simulink model "All_Car_Models"  (R2018b)
settings: Solver=VariableStepAuto  StartTime=0.0  StopTime=10.0  RelTol=1e-3
values from neighbouring files (symbols this model uses):
  a = 1.25    [SetCoefficients_FC.m]
  amplitude = 0.01    [SetCoefficients_FC.m]
  b = 1.4    [SetCoefficients_FC.m]
  c = 1.3    [SetCoefficients_FC.m]
  csc = 600    [SetCoefficients_FC.m]
  cse = 1200    [SetCoefficients_FC.m]
  d = 1.7    [SetCoefficients_FC.m]
  delay = (a+b)/v    [setSpeed.m]
  Fre_r = Fre*2*pi    [setSpeed.m]
  g = 9.81    [SetCoefficients_FC.m]
  HumpHight = 2    [SetCoefficients_FC.m]
  HumpLegnth = 20    [SetCoefficients_FC.m]
  I = 600    [SetCoefficients_FC.m]
  I_phi = 1000    [SetCoefficients_FC.m]
  I_theta = 600    [SetCoefficients_FC.m]
  ks =     [SetCoefficients.m]    (also in SetCoefficients_FC.m = 20000)
  ksSteel = 6.6e9    (= 6600000000)    [SetCoefficients_FC.m]
  ksstiff = 4e5    (= 400000)    [SetCoefficients_FC.m]
  kt =     [SetCoefficients.m]    (also in SetCoefficients_FC.m = 140000)
  m1 = 250    [SetCoefficients.m]    (also in SetCoefficients_FC.m)
  m2 =     [SetCoefficients.m]    (also in SetCoefficients_FC.m = 20)
  mb = 1000    [SetCoefficients_FC.m]
  mbh = mb/2    (= 500)    [SetCoefficients_FC.m]
  v_hump = v    [setSpeed.m]
  x1 = 0.2    [SetCoefficients_FC.m]
  x2 = 0.25    [SetCoefficients_FC.m]
  xt_Lim = 0.1    [SetCoefficients_FC.m]
(part 1 of 2)
settings Model: Creator=joebe  LastModifiedBy=joebe

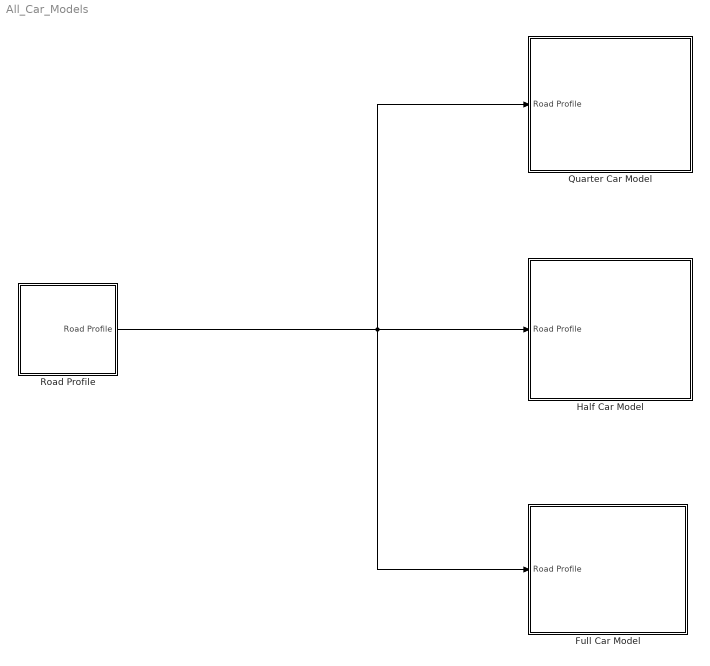
== system All_Car_Models ==
  Full Car Model : Subsystem
  Half Car Model : Subsystem
  Quarter Car Model : Subsystem
  Road Profile : Subsystem
  wires:
  Road Profile/1(Road Profile) -> Quarter Car Model/1(Road Profile), Full Car Model/1(Road Profile), Half Car Model/1(Road Profile)

== system All_Car_Models/Full Car Model ==
  Road Profile : Inport
  Bus Selector : BusSelector  OutputSignals=Body Vertical Motion.COM Displacement,Body Vertical Motion.COM Velocity,body pitch motion.Pitch Angle,body pitch motion.Pitch Velocity,Body Pitch motion.Roll Angle,Body Pitch motion.Roll Velocity
  Bus Selector1 : BusSelector  OutputSignals=Front Left Body Motion.Front Left Displacement,Front Right Body Motion.Front Right Displacement,Rear Left Body Motion.Rear Left Displacement,Rear Right Body Motion.Rear Right Displacement
  COM/Road displacement : Scope  NumInputPorts=2
  Full Car Model : Subsystem
  Pitch Angle : Scope
  Pitch Velocity : Scope
  Roll Angle : Scope
  Roll Velocity : Scope
  Tyre/COM displacements : Scope  NumInputPorts=5
  Vertical Displacement : Scope
  Vertical Velocity : Scope
  wires:
  Bus Selector1/2 -> Tyre/COM displacements/2  "<Front Right Displacement>"
  Bus Selector/3 -> Pitch Angle/1  "<Pitch Angle>"
  Full Car Model/1(Body Motion) -> Bus Selector/1
  Bus Selector/6 -> Roll Velocity/1  "<Roll Velocity>"
  Bus Selector/5 -> Roll Angle/1  "<Roll Angle>"
  Bus Selector/1 -> Vertical Displacement/1, Tyre/COM displacements/5, COM/Road displacement/1  "<COM Displacement>"
  Bus Selector/2 -> Vertical Velocity/1  "<COM Velocity>"
  Road Profile/1 -> Full Car Model/1(Road Profile), COM/Road displacement/2
  Bus Selector1/1 -> Tyre/COM displacements/1  "<Front Left Displacement>"
  Bus Selector1/3 -> Tyre/COM displacements/3  "<Rear Left Displacement>"
  Bus Selector/4 -> Pitch Velocity/1  "<Pitch Velocity>"
  Full Car Model/2(Body Section Motion) -> Bus Selector1/1
  Bus Selector1/4 -> Tyre/COM displacements/4  "<Rear Right Displacement>"

== system All_Car_Models/Half Car Model ==
  Road Profile : Inport
  1/2 Car Model : Subsystem
  1/2 Car Model Improved : Subsystem
  Body displacements : Scope  NumInputPorts=3
  Body displacements Improved model : Scope  NumInputPorts=3
  COM Body comparrison : Scope  NumInputPorts=2
  Demux{,1,3..4} (4 alike) : Demux
  wires:
  Demux1/3 -> Body displacements/2  "Rear Body displacement"
  Demux3/1 -> Body displacements Improved model/3, COM Body comparrison/2  "COM Displacement Improved Model"
  1/2 Car Model/2(Body Section motions) -> Demux1/1
  Demux/1 -> COM Body comparrison/1, Body displacements/3  "COM Displcameent Original Model"
  1/2 Car Model Improved/2(Body Section motions) -> Demux4/1
  Demux4/1 -> Body displacements Improved model/1  "Front Body Displacement"
  Road Profile/1 -> 1/2 Car Model/1(Road Profile), 1/2 Car Model Improved/1(Road Profile)
  1/2 Car Model Improved/1(Body Motion. (sb.sbd.theta,thetad)) -> Demux3/1
  Demux4/3 -> Body displacements Improved model/2  "Rear Body displacement"
  1/2 Car Model/1(Body Motion) -> Demux/1
  Demux1/1 -> Body displacements/1  "Front Body Displacement"

== system All_Car_Models/Quarter Car Model ==
  Road Profile : Inport
  Body Displacement : Scope
  Body Velocity : Scope
  Body Wheel and Road Displacement : Scope  NumInputPorts=3
  Demux : Demux  Outputs=2
  Demux1 : Demux  Outputs=2
  Quarter Car Model : Subsystem
  Wheel Displacement : Scope
  Wheel Velocity : Scope
  wires:
  Demux/2 -> Body Velocity/1  "Body Velcoity"
  Demux1/1 -> Body Wheel and Road Displacement/3, Wheel Displacement/1  "Wheel Displacement"
  Demux1/2 -> Wheel Velocity/1  "Wheel Velocity"
  Road Profile/1 -> Body Wheel and Road Displacement/2, Quarter Car Model/1(Road profile)
  Demux/1 -> Body Wheel and Road Displacement/1, Body Displacement/1  "Body Displacement"
  Quarter Car Model/1(Body Motion) -> Demux/1
  Quarter Car Model/2(Wheel Motion) -> Demux1/1

== system All_Car_Models/Road Profile ==
  Constant : Constant  Value=0
  Delay : TransportDelay  BufferSize=3072
  Delay1 : TransportDelay  BufferSize=3072
  Humpback bridge : Subsystem  mask{h=HumpHight, L=HumpLegnth, v=v_hump}
      mask prompts: h "humpback height (m)"; L "humpback length (m)"; v "vehicle speed (m/s)"
  Sine Wave : Sin  Amplitude=amplitude  Frequency=Fre_r  SampleTime=0
  Step Drop : Step  Time=2  After=-5  SampleTime=0
  Step Increase : Step  Time=2  SampleTime=0
  Road Profile : Outport
  wires:
  Humpback bridge/1(r) -> Delay1/1
  Sine Wave/1 -> Delay/1
  Delay1/1 -> Road Profile/1  "Road Profile"

== system All_Car_Models/Full Car Model/Full Car Model ==
  Road Profile : Inport
  Bus Creator : BusCreator  Inputs=4
  Bus Selector : BusSelector  OutputSignals=Front Left Body Motion,Rear Left Body Motion,Front Right Body Motion,Rear Right Body Motion
  Delay from front to rear wheels : TransportDelay  DelayTime=delay  BufferSize=3072
  Front Left Wheel Suspension model : Subsystem
  Front Right Suspension model : Subsystem
  Full Car Body Model : Subsystem
  Rear Left Wheel Suspension model : Subsystem
  Rear Right Suspension model : Subsystem
  Body Motion : Outport
  Body Section Motion : Outport  Port=2
  wires:
  Full Car Body Model/1(Body Motion) -> Body Motion/1
  Delay from front to rear wheels/1 -> Rear Right Suspension model/2(Road Profile), Rear Left Wheel Suspension model/2(Road Profile)
  Road Profile/1 -> Delay from front to rear wheels/1, Front Left Wheel Suspension model/2(Road Profile), Front Right Suspension model/2(Road Profile)
  Bus Selector/1 -> Front Left Wheel Suspension model/1(Body Motion)  "<Front Left Body Motion>"
  Front Left Wheel Suspension model/1(Front Left Suspension Force) -> Bus Creator/1  "Front Left  Suspension Force"
  Rear Right Suspension model/1(Rear Right Suspension Force) -> Bus Creator/3  "Rear Right  Suspension Force"
  Front Right Suspension model/1(Front Right Suspension Force) -> Bus Creator/4  "Front Right  Suspension Force"
  Bus Selector/3 -> Front Right Suspension model/1(Body Motion)  "<Front Right Body Motion>"
  Full Car Body Model/2(Body Section Motion) -> Bus Selector/1, Body Section Motion/1  "Body Section Motions"
  Bus Selector/2 -> Rear Left Wheel Suspension model/1(Body Motion)  "<Rear Left Body Motion>"
  Rear Left Wheel Suspension model/1(Rear Left Suspension Force) -> Bus Creator/2  "Rear Left  Suspension Force"
  Bus Selector/4 -> Rear Right Suspension model/1(Body Motion)  "<Rear Right Body Motion>"
  Bus Creator/1 -> Full Car Body Model/1(Suspention Forces)

== system All_Car_Models/Half Car Model/1//2 Car Model ==
  Road Profile : Inport
  1/2 car body model : Subsystem
  Delay from front to rear wheel : TransportDelay  DelayTime=delay  BufferSize=3072
  Front Wheel Suspention model : Subsystem
  Mux : Mux  Inputs=2
  Rear Wheel Suspention model : Subsystem
  Body Motion : Outport
  Body Section motions : Outport  Port=2
  wires:
  1/2 car body model/3(Rear Body Motion) -> Rear Wheel Suspention model/2(Body Motion), Mux/2  "Rear Body Motion"
  Front Wheel Suspention model/1(Front Suspention Force) -> 1/2 car body model/1(Front Suspention Force)  "Front Suspention Force"
  Rear Wheel Suspention model/1(Rear Suspention Force) -> 1/2 car body model/2(Rear Suspention Force)  "Rear Suspention Force"
  1/2 car body model/1(Front Body Motion) -> Front Wheel Suspention model/1(Body Motion), Mux/1  "Front Body Motion"
  1/2 car body model/2(Body Motion) -> Body Motion/1
  Road Profile/1 -> Front Wheel Suspention model/2(Road Profile), Delay from front to rear wheel/1
  Mux/1 -> Body Section motions/1
  Delay from front to rear wheel/1 -> Rear Wheel Suspention model/1(Road Profile)

== system All_Car_Models/Half Car Model/1//2 Car Model Improved ==
  note: Rear
  Road Profile : Inport
  1/2 car body model : Subsystem
  Delay from front to rear wheel2 : TransportDelay  DelayTime=delay  BufferSize=3072
  Front Wheel Suspension model : Subsystem
  Mux : Mux  Inputs=2
  Rear Wheel Suspension model : Subsystem
  Body Motion. (sb.sbd.theta,thetad) : Outport
  Body Section motions : Outport  Port=2
  wires:
  1/2 car body model/3(Rear Body Motion) -> Rear Wheel Suspension model/2(Body Motion), Mux/2  "Rear Body Motion"
  Front Wheel Suspension model/1(Fs) -> 1/2 car body model/1(Front Suspension Force)  "Front Suspension Force"
  Rear Wheel Suspension model/1(Fs) -> 1/2 car body model/2(Rear Suspension Force)  "Rear Suspension Force"
  1/2 car body model/1(Front Body Motion) -> Mux/1, Front Wheel Suspension model/1(Body Motion)  "Front Body Motion"
  1/2 car body model/2(Body Motion) -> Body Motion. (sb.sbd.theta,thetad)/1  "Body Motion. (sb.sbd.theta,thetad)"
  Road Profile/1 -> Delay from front to rear wheel2/1, Front Wheel Suspension model/2(Road Profile)
  Mux/1 -> Body Section motions/1
  Delay from front to rear wheel2/1 -> Rear Wheel Suspension model/1(Road Profile)

== system All_Car_Models/Quarter Car Model/Quarter Car Model ==
  Road profile : Inport
  Body Model : Subsystem
  Suspention Model : Subsystem
  Wheel Model : Subsystem
  Body Motion : Outport
  Wheel Motion : Outport  Port=2
  wires:
  Suspention Model/1(Suspention Force) -> Body Model/1("Suspention Force "), Wheel Model/2(Suspention force)  "Suspention Force"
  Wheel Model/1(Wheel Motion) -> Wheel Motion/1, Suspention Model/1(Wheel Motion)  "Wheel Motion"
  Body Model/1(Body Motion) -> Body Motion/1, Suspention Model/2(Body Motion)  "Body Motion"
  Road profile/1 -> Wheel Model/1(Road Profile)  "Road Profile"

== system All_Car_Models/Road Profile/Humpback bridge ==
  Add : Sum  Inputs=+-
  Constant : Constant  Value=h/2
  Product : Product
  Product1 : Product
  Sine Wave : Sin  Amplitude=h/2  Frequency=2*pi*v_hump/L  Phase=pi/2  SampleTime=0
  Step : Step  Time=0  SampleTime=0
  Step1 : Step  Time=L/v_hump  Before=1  After=0  SampleTime=0
  r : Outport
  wires:
  Constant/1 -> Add/1
  Sine Wave/1 -> Add/2
  Add/1 -> Product/1
  Step/1 -> Product/2
  Product/1 -> Product1/1
  Step1/1 -> Product1/2
  Product1/1 -> r/1

== system All_Car_Models/Full Car Model/Full Car Model/Front Left Wheel Suspension model ==
  Body Motion : Inport
  Road Profile : Inport  Port=2
  Suspention Model : Subsystem
  Wheel Model : Subsystem
  Front Left Suspension Force : Outport
  wires:
  Wheel Model/1(Wheel Motion) -> Suspention Model/1(Wheel Motion)  "s2.s2d"
  Road Profile/1 -> Wheel Model/2(Road Profile)
  Suspention Model/1(Suspension Force) -> Front Left Suspension Force/1, Wheel Model/1(Suspension force)
  Body Motion/1 -> Suspention Model/2(Body Motion)

== system All_Car_Models/Full Car Model/Full Car Model/Front Right Suspension model ==
  Body Motion : Inport
  Road Profile : Inport  Port=2
  Suspension Model : Subsystem
  Wheel Model : Subsystem
  Front Right Suspension Force : Outport
  wires:
  Wheel Model/1(Wheel Motion) -> Suspension Model/1(Wheel Motion)  "s2.s2d"
  Road Profile/1 -> Wheel Model/2(Road Profile)
  Suspension Model/1(Suspension Force) -> Front Right Suspension Force/1, Wheel Model/1(Suspension force)
  Body Motion/1 -> Suspension Model/2(Body Motion)

== system All_Car_Models/Full Car Model/Full Car Model/Full Car Body Model ==
  Suspention Forces : Inport
  Bus Creator : BusCreator  Inputs=3
  Bus Creator1 : BusCreator  Inputs=4
  Bus Selector : BusSelector  OutputSignals=|
      | Front Right 
      | Suspension Force,Front Left 
      | Suspension Force,Rear Right 
      | Suspension Force,Rear Left 
      | Suspension Force
  Car Pitch Motion : Subsystem
  Car Roll Motion1 : Subsystem
  Car Vertical Motion : Subsystem
  Front Left Body Motion : Subsystem
  "Front Right Body Motion " : Subsystem
  Rear Left Body Motion : Subsystem
  Rear Right Body Motion : Subsystem
  Body Motion : Outport
  Body Section Motion : Outport  Port=2
  wires:
  Bus Selector/1 -> Car Roll Motion1/1(Front Right Suspention force), Car Pitch Motion/1(Front Right Suspention force), Car Vertical Motion/1(Front Right Suspention force)  "<Front Right  Suspension Force>"
  Bus Selector/2 -> Car Roll Motion1/2(Front Left Suspention force), Car Pitch Motion/2(Front Left Suspention force), Car Vertical Motion/2(Front Left Suspention force)  "<Front Left  Suspension Force>"
  Bus Selector/3 -> Car Roll Motion1/3(Rear Right Suspention force), Car Pitch Motion/3(Rear Right Suspention force), Car Vertical Motion/3(Rear Right Suspention force)  "<Rear Right  Suspension Force>"
  Car Vertical Motion/1(Body Vertical Motion) -> Bus Creator/1, Rear Right Body Motion/1(Body Vertical Motion), Rear Left Body Motion/1(Body Vertical Motion), "Front Right Body Motion "/1(Body Vertical Motion), Front Left Body Motion/1(Body Vertical Motion)
  Bus Selector/4 -> Car Roll Motion1/4(Rear Left Suspention force), Car Pitch Motion/4(Rear Left Suspention force), Car Vertical Motion/4(Rear Left Suspention force)  "<Rear Left  Suspension Force>"
  Car Roll Motion1/1(Body Roll Motion) -> Front Left Body Motion/3(Body Roll Motion), "Front Right Body Motion "/3(Body Roll Motion), Rear Left Body Motion/3(Body Roll Motion), Bus Creator/3, Rear Right Body Motion/3(Body Roll Motion)
  Car Pitch Motion/1(body pitch motion) -> Front Left Body Motion/2(Body Pitch Motion), "Front Right Body Motion "/2(Body Pitch Motion), Bus Creator/2, Rear Right Body Motion/2(Body Pitch Motion), Rear Left Body Motion/2(Body Pitch Motion)
  Bus Creator/1 -> Body Motion/1
  Bus Creator1/1 -> Body Section Motion/1
  Front Left Body Motion/1(Front Left Body Motion) -> Bus Creator1/1
  "Front Right Body Motion "/1(Front Right Body Motion) -> Bus Creator1/2
  Rear Left Body Motion/1(Rear Left Body Motion) -> Bus Creator1/3
  Rear Right Body Motion/1(Rear Right Body Motion) -> Bus Creator1/4
  Suspention Forces/1 -> Bus Selector/1

== system All_Car_Models/Full Car Model/Full Car Model/Rear Left Wheel Suspension model ==
  Body Motion : Inport
  Road Profile : Inport  Port=2
  Suspension Model : Subsystem
  Wheel Model : Subsystem
  Rear Left Suspension Force : Outport
  wires:
  Wheel Model/1(Wheel Motion) -> Suspension Model/1(Wheel Motion)  "s2.s2d"
  Road Profile/1 -> Wheel Model/2(Road Profile)
  Suspension Model/1(Suspension Force) -> Rear Left Suspension Force/1, Wheel Model/1(Suspension force)
  Body Motion/1 -> Suspension Model/2(Body Motion)

== system All_Car_Models/Full Car Model/Full Car Model/Rear Right Suspension model ==
  Body Motion : Inport
  Road Profile : Inport  Port=2
  Suspention Model : Subsystem
  Wheel Model : Subsystem
  Rear Right Suspension Force : Outport
  wires:
  Wheel Model/1(Wheel Motion) -> Suspention Model/1(Wheel Motion)  "s2.s2d"
  Road Profile/1 -> Wheel Model/2(Road Profile)
  Suspention Model/1(Suspension Force) -> Rear Right Suspension Force/1, Wheel Model/1(Suspension force)
  Body Motion/1 -> Suspention Model/2(Body Motion)

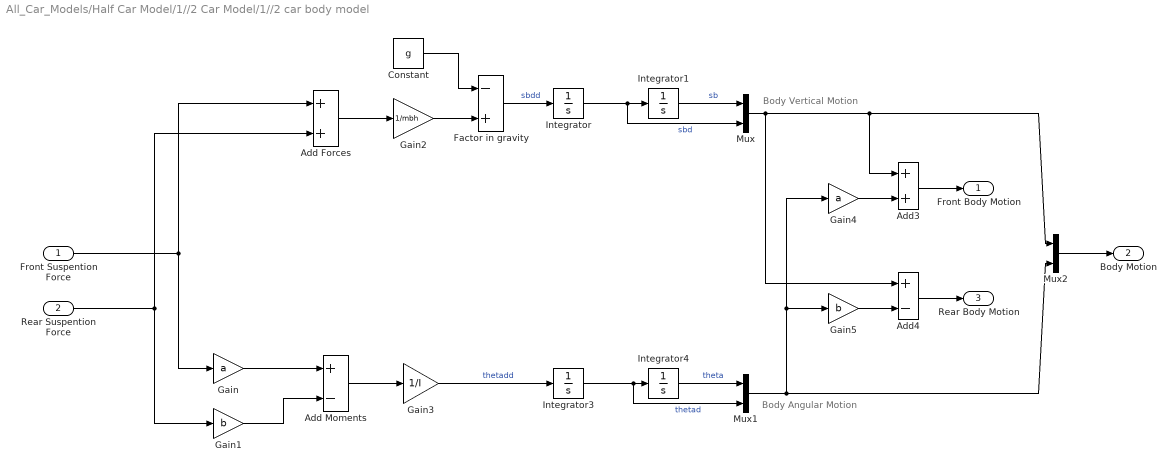
== system All_Car_Models/Half Car Model/1//2 Car Model/1//2 car body model ==
  note: Body Angular Motion
  note: Body Vertical Motion
  Front Suspention Force : Inport
  Rear Suspention Force : Inport  Port=2
  Add Forces : Sum
  Add Moments : Sum  Inputs=+-
  Add3 : Sum
  Add4 : Sum  Inputs=+-
  Constant : Constant  Value=g
  Factor in gravity : Sum  Inputs=-+
  Gain : Gain  Gain=a
  Gain1 : Gain  Gain=b
  Gain2 : Gain  Gain=1/mbh
  Gain3 : Gain  Gain=1/I
  Gain4 : Gain  Gain=a
  Gain5 : Gain  Gain=b
  Integrator : Integrator
  Integrator1 : Integrator  InitialCondition=-0.142
  Integrator3 : Integrator
  Integrator4 : Integrator  InitialCondition=-6e-3
  Mux : Mux  Inputs=2
  Mux1 : Mux  Inputs=2
  Mux2 : Mux  Inputs=2
  Front Body Motion : Outport
  Body Motion : Outport  Port=2
  Rear Body Motion : Outport  Port=3
  wires:
  Add Forces/1 -> Gain2/1
  Mux1/1 -> Gain4/1, Gain5/1, Mux2/2
  Integrator3/1 -> Mux1/2, Integrator4/1  "thetad"
  Add Moments/1 -> Gain3/1
  Gain3/1 -> Integrator3/1  "thetadd"
  Mux2/1 -> Body Motion/1
  Gain2/1 -> Factor in gravity/2
  Mux/1 -> Add4/1, Add3/1, Mux2/1
  Gain4/1 -> Add3/2
  Gain/1 -> Add Moments/1
  Integrator4/1 -> Mux1/1  "theta"
  Integrator/1 -> Mux/2, Integrator1/1  "sbd"
  Rear Suspention Force/1 -> Add Forces/2, Gain1/1
  Front Suspention Force/1 -> Gain/1, Add Forces/1
  Integrator1/1 -> Mux/1  "sb"
  Gain1/1 -> Add Moments/2
  Add3/1 -> Front Body Motion/1
  Gain5/1 -> Add4/2
  Constant/1 -> Factor in gravity/1
  Factor in gravity/1 -> Integrator/1  "sbdd"
  Add4/1 -> Rear Body Motion/1

== system All_Car_Models/Half Car Model/1//2 Car Model/Front Wheel Suspention model ==
  Body Motion : Inport
  Road Profile : Inport  Port=2
  Suspention Model : Subsystem
  Wheel Model : Subsystem
  Front Suspention Force : Outport
  wires:
  Wheel Model/1(Wheel Motion) -> Suspention Model/1(Wheel Motion)
  Road Profile/1 -> Wheel Model/2(Road Profile)
  Suspention Model/1(Suspention Force) -> Front Suspention Force/1, Wheel Model/1(Suspention force)
  Body Motion/1 -> Suspention Model/2(Body Motion)

== system All_Car_Models/Half Car Model/1//2 Car Model/Rear Wheel Suspention model ==
  Road Profile : Inport
  Body Motion : Inport  Port=2
  Suspention Model : Subsystem
  Wheel Model : Subsystem
  Rear Suspention Force : Outport
  wires:
  Wheel Model/1(Wheel Motion) -> Suspention Model/1(Wheel Motion)  "s2.s2d"
  Road Profile/1 -> Wheel Model/2(Road Profile)
  Suspention Model/1(Suspention Force) -> Rear Suspention Force/1, Wheel Model/1(Suspention force)
  Body Motion/1 -> Suspention Model/2(Body Motion)

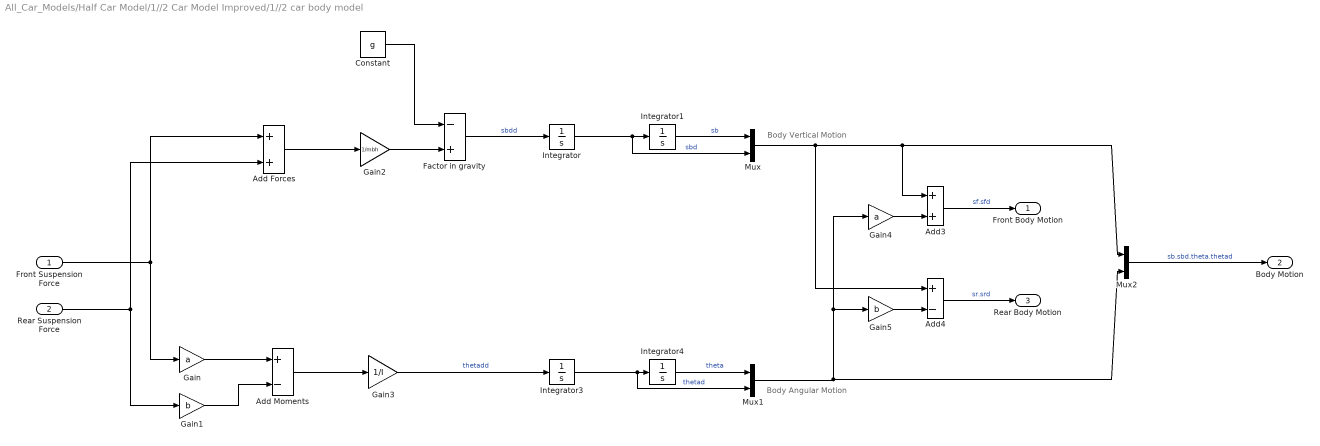
== system All_Car_Models/Half Car Model/1//2 Car Model Improved/1//2 car body model ==
  note: Body Angular Motion
  note: Body Vertical Motion
  Front Suspension Force : Inport
  Rear Suspension Force : Inport  Port=2
  Add Forces : Sum
  Add Moments : Sum  Inputs=+-
  Add3 : Sum
  Add4 : Sum  Inputs=+-
  Constant : Constant  Value=g
  Factor in gravity : Sum  Inputs=-+
  Gain : Gain  Gain=a
  Gain1 : Gain  Gain=b
  Gain2 : Gain  Gain=1/mbh
  Gain3 : Gain  Gain=1/I
  Gain4 : Gain  Gain=a
  Gain5 : Gain  Gain=b
  Integrator : Integrator
  Integrator1 : Integrator  InitialCondition=-0.142
  Integrator3 : Integrator
  Integrator4 : Integrator  InitialCondition=-6e-3
  Mux : Mux  Inputs=2
  Mux1 : Mux  Inputs=2
  Mux2 : Mux  Inputs=2
  Front Body Motion : Outport
  Body Motion : Outport  Port=2
  Rear Body Motion : Outport  Port=3
  wires:
  Add Forces/1 -> Gain2/1
  Mux1/1 -> Gain4/1, Gain5/1, Mux2/2
  Integrator3/1 -> Mux1/2, Integrator4/1  "thetad"
  Add Moments/1 -> Gain3/1
  Gain3/1 -> Integrator3/1  "thetadd"
  Mux2/1 -> Body Motion/1  "sb.sbd.theta.thetad"
  Gain2/1 -> Factor in gravity/2
  Mux/1 -> Add4/1, Add3/1, Mux2/1
  Gain4/1 -> Add3/2
  Gain/1 -> Add Moments/1
  Integrator4/1 -> Mux1/1  "theta"
  Integrator/1 -> Mux/2, Integrator1/1  "sbd"
  Rear Suspension Force/1 -> Add Forces/2, Gain1/1
  Front Suspension Force/1 -> Gain/1, Add Forces/1
  Integrator1/1 -> Mux/1  "sb"
  Gain1/1 -> Add Moments/2
  Add3/1 -> Front Body Motion/1  "sf.sfd"
  Gain5/1 -> Add4/2
  Constant/1 -> Factor in gravity/1
  Factor in gravity/1 -> Integrator/1  "sbdd"
  Add4/1 -> Rear Body Motion/1  "sr.srd"

== system All_Car_Models/Half Car Model/1//2 Car Model Improved/Front Wheel Suspension model ==
  Body Motion : Inport
  Road Profile : Inport  Port=2
  Suspension Model : Subsystem
  Wheel Model : Subsystem
  Fs : Outport
  wires:
  Wheel Model/1(Wheel Motion) -> Suspension Model/1(Wheel Motion)  "s2.s2d"
  Road Profile/1 -> Wheel Model/2(Road Profile)
  Suspension Model/1(Suspension Force) -> Fs/1, Wheel Model/1(Suspension force)
  Body Motion/1 -> Suspension Model/2(Body Motion)

== system All_Car_Models/Half Car Model/1//2 Car Model Improved/Rear Wheel Suspension model ==
  Road Profile : Inport
  Body Motion : Inport  Port=2
  Suspention Model : Subsystem
  Wheel Model : Subsystem
  Fs : Outport
  wires:
  Wheel Model/1(Wheel Motion) -> Suspention Model/1(Wheel Motion)  "s2.s2d"
  Road Profile/1 -> Wheel Model/2(Road Profile)
  Suspention Model/1(Suspension Force) -> Fs/1, Wheel Model/1(Suspention force)
  Body Motion/1 -> Suspention Model/2(Body Motion)

== system All_Car_Models/Quarter Car Model/Quarter Car Model/Body Model ==
  note: Body Velocity
  note: Body displacement
  note: Body Acceleration
  "Suspention Force " : Inport
  Acceleration due to gravity : Constant  Value=g*m1
  Add : Sum  Inputs=-+
  Body mass : Gain  Gain=1/m1
  Integrator : Integrator
  Integrator1 : Integrator
  Mux : Mux  Inputs=2
  Body Motion : Outport
  wires:
  "Suspention Force "/1 -> Add/2
  Integrator/1 -> Mux/2, Integrator1/1
  Add/1 -> Body mass/1
  Acceleration due to gravity/1 -> Add/1
  Integrator1/1 -> Mux/1
  Mux/1 -> Body Motion/1
  Body mass/1 -> Integrator/1

== system All_Car_Models/Quarter Car Model/Quarter Car Model/Suspention Model ==
  note: s1.s1d
  note: s2.s2d
  Wheel Motion : Inport
  Body Motion : Inport  Port=2
  " " : Sum  Inputs=+-
  " " : Sum  Inputs=+-
  1-D Lookup Table : Lookup_n-D  NumberOfTableDimensions=1  BreakpointsForDimension1=[-x2 -x1 x1 x2]  Table=[-(ksstiff*(x2-x1)+ks*x1) -x1*ks x1*ks (ksstiff*(x2-x1)+ks*x1)]  InternalRulePriority=Speed  RndMeth=Simplest  InputSameDT=on
  1-D Lookup Table1 : Lookup_n-D  NumberOfTableDimensions=1  BreakpointsForDimension1=[-10 0 10]  Table=[-10*cse 0 10*csc]  InternalRulePriority=Speed  RndMeth=Simplest  InputSameDT=on
  Add suspention forces : Sum
  Demux : Demux  Outputs=2
  Demux1 : Demux  Outputs=2
  Suspention Force : Outport
  wires:
  Demux1/2 -> " "/2  "s1d"
  " "/1 -> 1-D Lookup Table/1  "s1-s2"
  Demux1/1 -> " "/2  "s1"
  1-D Lookup Table1/1 -> Add suspention forces/2
  1-D Lookup Table/1 -> Add suspention forces/1
  Demux/1 -> " "/1  "s2"
  Demux/2 -> " "/1  "s2d"
  Body Motion/1 -> Demux1/1
  " "/1 -> 1-D Lookup Table1/1  "s1d-s2d"
  Add suspention forces/1 -> Suspention Force/1
  Wheel Motion/1 -> Demux/1

== system All_Car_Models/Quarter Car Model/Quarter Car Model/Wheel Model ==
  Road Profile : Inport
  Suspention force : Inport  Port=2
  Acceleration due to gravity : Constant  Value=g*m2
  Add : Sum  Inputs=+--
  Compression only : Saturate  UpperLimit=inf  LowerLimit=0
  Gain : Gain  Gain=1/m2
  Gain1 : Gain  Gain=kt
  Integrator : Integrator
  Integrator1 : Integrator
  Mux : Mux  Inputs=2
  tyre extention/conpression : Sum  Inputs=+-
  Wheel Motion : Outport
  wires:
  Integrator1/1 -> tyre extention/conpression/2, Mux/1  "Wheel Displacement"
  Integrator/1 -> Mux/2, Integrator1/1  "Wheel Velocity"
  Add/1 -> Gain/1
  Gain1/1 -> Add/1  "Tyre Force"
  Road Profile/1 -> tyre extention/conpression/1
  Mux/1 -> Wheel Motion/1  "s2.s2d"
  Acceleration due to gravity/1 -> Add/3
  Suspention force/1 -> Add/2
  Gain/1 -> Integrator/1  "Wheel Acceleration"
  tyre extention/conpression/1 -> Gain1/1  "r-s2"

== system All_Car_Models/Full Car Model/Full Car Model/Front Left Wheel Suspension model/Suspention Model ==
  note: s1.s1d
  note: s2.s2d
  Wheel Motion : Inport
  Body Motion : Inport  Port=2
  " " : Sum  Inputs=+-
  " " : Sum  Inputs=+-
  Add Suspension forces : Sum
  Bus Selector : BusSelector  OutputSignals=Front Left Displacement,Front Left Velocity
  Demux : Demux  Outputs=2
  Suspension Damping Coefficient : Lookup_n-D  NumberOfTableDimensions=1  BreakpointsForDimension1=[-10 0 10]  Table=[-10*cse 0 10*csc]  InternalRulePriority=Speed  RndMeth=Simplest  InputSameDT=on
  Suspension Spring Coefficient : Lookup_n-D  NumberOfTableDimensions=1  BreakpointsForDimension1=([0 x1 x2 2*x2])  Table=([0 ks*x1 ksstiff*(x2-x1)-(ks*x1) ksSteel*x2-(ksstiff*(x2-x1)-(ks*x1))])  InternalRulePriority=Speed  RndMeth=Simplest  InputSameDT=on
  Suspension Force : Outport
  wires:
  Bus Selector/2 -> " "/2  "<Front Left Velocity>"
  " "/1 -> Suspension Spring Coefficient/1  "s1-s2"
  Bus Selector/1 -> " "/2  "<Front Left Displacement>"
  Suspension Damping Coefficient/1 -> Add Suspension forces/2
  Suspension Spring Coefficient/1 -> Add Suspension forces/1
  Demux/1 -> " "/1  "Front Left Wheel Displacment"
  Demux/2 -> " "/1  "Front Left Wheel Velocity"
  Body Motion/1 -> Bus Selector/1
  " "/1 -> Suspension Damping Coefficient/1  "s1d-s2d"
  Add Suspension forces/1 -> Suspension Force/1
  Wheel Motion/1 -> Demux/1

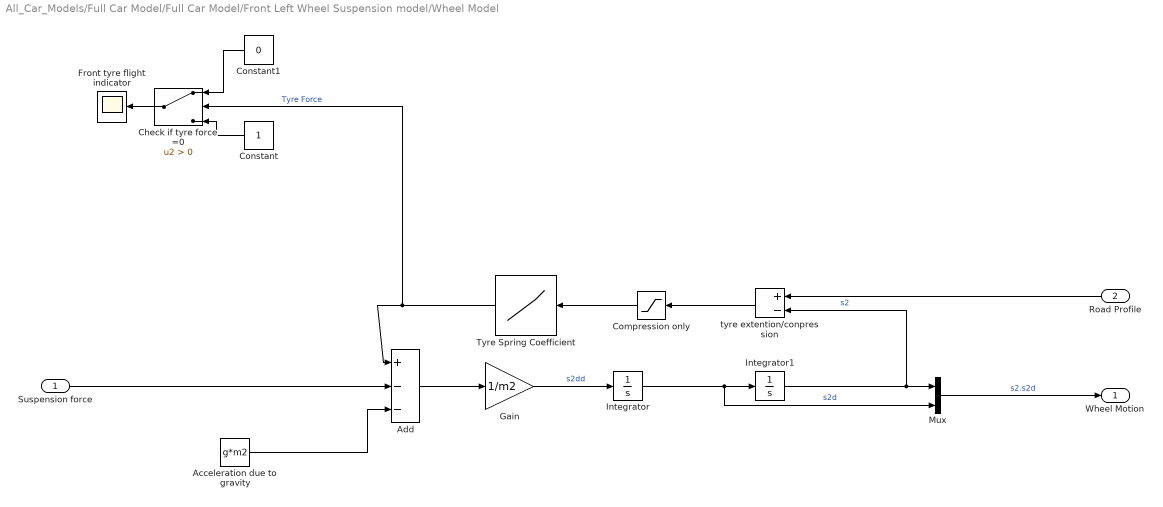
== system All_Car_Models/Full Car Model/Full Car Model/Front Left Wheel Suspension model/Wheel Model ==
  Suspension force : Inport
  Road Profile : Inport  Port=2
  Acceleration due to gravity : Constant  Value=g*m2
  Add : Sum  Inputs=+--
  Check if tyre force =0 : Switch  Criteria=u2 > Threshold
  Compression only : Saturate  UpperLimit=inf  LowerLimit=0
  Constant : Constant
  Constant1 : Constant  Value=0
  Front tyre flight indicator : Scope
  Gain : Gain  Gain=1/m2
  Integrator : Integrator
  Integrator1 : Integrator  InitialCondition=-2.23e-02
  Mux : Mux  Inputs=2
  Tyre Spring Coefficient : Lookup_n-D  NumberOfTableDimensions=1  BreakpointsForDimension1=[0 xt_Lim 2*xt_Lim]  Table=[0 xt_Lim*kt ksSteel*2*xt_Lim]  InternalRulePriority=Speed  RndMeth=Simplest  InputSameDT=on
  tyre extention/conpression : Sum  Inputs=+-
  Wheel Motion : Outport
  wires:
  Integrator1/1 -> Mux/1, tyre extention/conpression/2  "s2"
  Integrator/1 -> Mux/2, Integrator1/1  "s2d"
  Add/1 -> Gain/1
  Tyre Spring Coefficient/1 -> Check if tyre force =0/2, Add/1  "Tyre Force"
  Road Profile/1 -> tyre extention/conpression/1
  Mux/1 -> Wheel Motion/1  "s2.s2d"
  Acceleration due to gravity/1 -> Add/3
  Suspension force/1 -> Add/2
  Gain/1 -> Integrator/1  "s2dd"
  tyre extention/conpression/1 -> Compression only/1
  Compression only/1 -> Tyre Spring Coefficient/1
  Check if tyre force =0/1 -> Front tyre flight indicator/1
  Constant1/1 -> Check if tyre force =0/1
  Constant/1 -> Check if tyre force =0/3

== system All_Car_Models/Full Car Model/Full Car Model/Front Right Suspension model/Suspension Model ==
  note: s1.s1d
  note: s2.s2d
  Wheel Motion : Inport
  Body Motion : Inport  Port=2
  " " : Sum  Inputs=+-
  " " : Sum  Inputs=+-
  Add Suspension forces : Sum
  Bus Selector : BusSelector  OutputSignals=Front Right Displacement,Front Right Velocity
  Demux : Demux  Outputs=2
  Spring Coefficient : Lookup_n-D  NumberOfTableDimensions=1  BreakpointsForDimension1=([0 x1 x2 2*x2])  Table=([0 ks*x1 ksstiff*(x2-x1)-(ks*x1) ksSteel*x2-(ksstiff*(x2-x1)-(ks*x1))])  InternalRulePriority=Speed  RndMeth=Simplest  InputSameDT=on
  Suspension Damping Coefficient : Lookup_n-D  NumberOfTableDimensions=1  BreakpointsForDimension1=[-10 0 10]  Table=[-10*cse 0 10*csc]  InternalRulePriority=Speed  RndMeth=Simplest  InputSameDT=on
  Suspension Force : Outport
  wires:
  Bus Selector/2 -> " "/2  "<Front Right Velocity>"
  " "/1 -> Spring Coefficient/1  "s1-s2"
  Bus Selector/1 -> " "/2  "<Front Right Displacement>"
  Suspension Damping Coefficient/1 -> Add Suspension forces/2
  Spring Coefficient/1 -> Add Suspension forces/1
  Demux/1 -> " "/1  "Front Right Wheel Displacements"
  Demux/2 -> " "/1  "Front Left Wheel Velocity"
  Body Motion/1 -> Bus Selector/1
  " "/1 -> Suspension Damping Coefficient/1  "s1d-s2d"
  Add Suspension forces/1 -> Suspension Force/1
  Wheel Motion/1 -> Demux/1

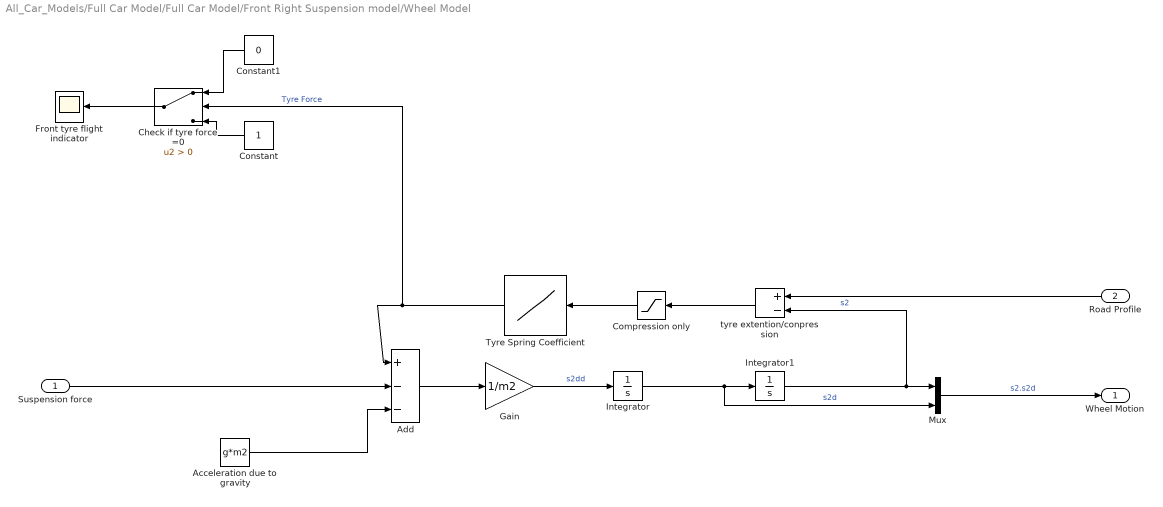
== system All_Car_Models/Full Car Model/Full Car Model/Front Right Suspension model/Wheel Model ==
  Suspension force : Inport
  Road Profile : Inport  Port=2
  Acceleration due to gravity : Constant  Value=g*m2
  Add : Sum  Inputs=+--
  Check if tyre force =0 : Switch  Criteria=u2 > Threshold
  Compression only : Saturate  UpperLimit=inf  LowerLimit=0
  Constant : Constant
  Constant1 : Constant  Value=0
  Front tyre flight indicator : Scope
  Gain : Gain  Gain=1/m2
  Integrator : Integrator
  Integrator1 : Integrator  InitialCondition=-1.76e-02
  Mux : Mux  Inputs=2
  Tyre Spring Coefficient : Lookup_n-D  NumberOfTableDimensions=1  BreakpointsForDimension1=[0 xt_Lim 2*xt_Lim]  Table=[0 xt_Lim*kt ksSteel*2*xt_Lim]  InternalRulePriority=Speed  RndMeth=Simplest  InputSameDT=on
  tyre extention/conpression : Sum  Inputs=+-
  Wheel Motion : Outport
  wires:
  Integrator1/1 -> Mux/1, tyre extention/conpression/2  "s2"
  Integrator/1 -> Mux/2, Integrator1/1  "s2d"
  Add/1 -> Gain/1
  Tyre Spring Coefficient/1 -> Check if tyre force =0/2, Add/1  "Tyre Force"
  Road Profile/1 -> tyre extention/conpression/1
  Mux/1 -> Wheel Motion/1  "s2.s2d"
  Acceleration due to gravity/1 -> Add/3
  Suspension force/1 -> Add/2
  Gain/1 -> Integrator/1  "s2dd"
  tyre extention/conpression/1 -> Compression only/1
  Compression only/1 -> Tyre Spring Coefficient/1
  Check if tyre force =0/1 -> Front tyre flight indicator/1
  Constant1/1 -> Check if tyre force =0/1
  Constant/1 -> Check if tyre force =0/3

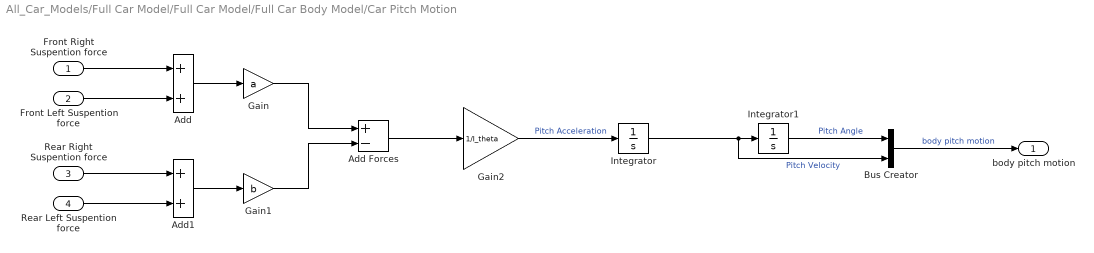
== system All_Car_Models/Full Car Model/Full Car Model/Full Car Body Model/Car Pitch Motion ==
  Front Right Suspention force : Inport
  Front Left Suspention force : Inport  Port=2
  Rear Right Suspention force : Inport  Port=3
  Rear Left Suspention force : Inport  Port=4
  Add : Sum
  Add Forces : Sum  Inputs=+-
  Add1 : Sum
  Bus Creator : BusCreator  Inputs=2
  Gain : Gain  Gain=a
  Gain1 : Gain  Gain=b
  Gain2 : Gain  Gain=1/I_theta
  Integrator : Integrator
  Integrator1 : Integrator  InitialCondition=-6e-03
  body pitch motion : Outport
  wires:
  Gain/1 -> Add Forces/1
  Gain1/1 -> Add Forces/2
  Gain2/1 -> Integrator/1  "Pitch Acceleration"
  Add1/1 -> Gain1/1
  Add Forces/1 -> Gain2/1
  Integrator/1 -> Bus Creator/2, Integrator1/1  "Pitch Velocity"
  Rear Right Suspention force/1 -> Add1/1
  Add/1 -> Gain/1
  Integrator1/1 -> Bus Creator/1  "Pitch Angle"
  Front Right Suspention force/1 -> Add/1
  Bus Creator/1 -> body pitch motion/1  "body pitch motion"
  Front Left Suspention force/1 -> Add/2
  Rear Left Suspention force/1 -> Add1/2

== system All_Car_Models/Full Car Model/Full Car Model/Full Car Body Model/Car Roll Motion1 ==
  Front Right Suspention force : Inport
  Front Left Suspention force : Inport  Port=2
  Rear Right Suspention force : Inport  Port=3
  Rear Left Suspention force : Inport  Port=4
  Add : Sum
  Add1 : Sum
  Add2 : Sum  Inputs=-+
  Bus Creator : BusCreator  Inputs=2
  Gain : Gain  Gain=d
  Gain1 : Gain  Gain=c
  Gain2 : Gain  Gain=1/I_phi
  Integrator : Integrator
  Integrator1 : Integrator  InitialCondition=-1.246e-02
  Body Roll Motion : Outport
  wires:
  Gain/1 -> Add2/1
  Gain1/1 -> Add2/2
  Gain2/1 -> Integrator/1  "Roll Acceleration"
  Add1/1 -> Gain1/1
  Add2/1 -> Gain2/1
  Integrator/1 -> Bus Creator/2, Integrator1/1  "Roll Velocity"
  Add/1 -> Gain/1
  Integrator1/1 -> Bus Creator/1  "Roll Angle"
  Front Right Suspention force/1 -> Add/1
  Bus Creator/1 -> Body Roll Motion/1  "Body Pitch motion"
  Rear Left Suspention force/1 -> Add1/2
  Rear Right Suspention force/1 -> Add/2
  Front Left Suspention force/1 -> Add1/1

== system All_Car_Models/Full Car Model/Full Car Model/Full Car Body Model/Car Vertical Motion ==
  Front Right Suspention force : Inport
  Front Left Suspention force : Inport  Port=2
  Rear Right Suspention force : Inport  Port=3
  Rear Left Suspention force : Inport  Port=4
  Add : Sum  Inputs=++++
  Add1 : Sum  Inputs=-+
  Bus Creator : BusCreator  Inputs=2
  Constant : Constant  Value=g
  Gain : Gain  Gain=1/mb
  Integrator : Integrator
  Integrator1 : Integrator  InitialCondition=-1.445e-01
  Body Vertical Motion : Outport
  wires:
  Constant/1 -> Add1/1
  Add1/1 -> Integrator/1  "COM Acceleration"
  Add/1 -> Gain/1
  Integrator/1 -> Bus Creator/2, Integrator1/1  "COM Velocity"
  Integrator1/1 -> Bus Creator/1  "COM Displacement"
  Rear Right Suspention force/1 -> Add/3
  Gain/1 -> Add1/2
  Bus Creator/1 -> Body Vertical Motion/1  "Body Vertical Motion"
  Front Left Suspention force/1 -> Add/2
  Front Right Suspention force/1 -> Add/1
  Rear Left Suspention force/1 -> Add/4

== system All_Car_Models/Full Car Model/Full Car Model/Full Car Body Model/Front Left Body Motion ==
  Body Vertical Motion : Inport
  Body Pitch Motion : Inport  Port=2
  Body Roll Motion : Inport  Port=3
  Add : Sum  Inputs=+++
  Bus Creator : BusCreator  Inputs=2
  Demux : Demux  Outputs=2
  Gain : Gain  Gain=a
  Gain1 : Gain  Gain=c
  Front Left Body Motion : Outport
  wires:
  Gain1/1 -> Add/3
  Body Pitch Motion/1 -> Gain/1
  Gain/1 -> Add/2
  Body Vertical Motion/1 -> Add/1
  Add/1 -> Demux/1
  Demux/1 -> Bus Creator/1  "Front Left Displacement"
  Demux/2 -> Bus Creator/2  "Front Left Velocity"
  Bus Creator/1 -> Front Left Body Motion/1  "Front Left Body Motion"
  Body Roll Motion/1 -> Gain1/1

== system All_Car_Models/Full Car Model/Full Car Model/Full Car Body Model/Front Right Body Motion  ==
  Body Vertical Motion : Inport
  Body Pitch Motion : Inport  Port=2
  Body Roll Motion : Inport  Port=3
  Add : Sum  Inputs=++-
  Bus Creator : BusCreator  Inputs=2
  Demux : Demux  Outputs=2
  Gain : Gain  Gain=a
  Gain1 : Gain  Gain=d
  Front Right Body Motion : Outport
  wires:
  Body Roll Motion/1 -> Gain1/1
  Gain1/1 -> Add/3
  Body Pitch Motion/1 -> Gain/1
  Gain/1 -> Add/2
  Body Vertical Motion/1 -> Add/1
  Demux/1 -> Bus Creator/1  "Front Right Displacement"
  Demux/2 -> Bus Creator/2  "Front Right Velocity"
  Add/1 -> Demux/1
  Bus Creator/1 -> Front Right Body Motion/1  "Front Right Body Motion"

== system All_Car_Models/Full Car Model/Full Car Model/Full Car Body Model/Rear Left Body Motion ==
  Body Vertical Motion : Inport
  Body Pitch Motion : Inport  Port=2
  Body Roll Motion : Inport  Port=3
  Add : Sum  Inputs=+-+
  Bus Creator : BusCreator  Inputs=2
  Demux : Demux  Outputs=2
  Gain : Gain  Gain=b
  Gain1 : Gain  Gain=c
  Rear Left Body Motion : Outport
  wires:
  Body Roll Motion/1 -> Gain1/1
  Gain1/1 -> Add/3
  Body Pitch Motion/1 -> Gain/1
  Gain/1 -> Add/2
  Body Vertical Motion/1 -> Add/1
  Demux/1 -> Bus Creator/1  "Rear Left Displacement"
  Demux/2 -> Bus Creator/2  "Rear Left Velocity"
  Add/1 -> Demux/1
  Bus Creator/1 -> Rear Left Body Motion/1  "Rear Left Body Motion"

== system All_Car_Models/Full Car Model/Full Car Model/Full Car Body Model/Rear Right Body Motion ==
  Body Vertical Motion : Inport
  Body Pitch Motion : Inport  Port=2
  Body Roll Motion : Inport  Port=3
  Add : Sum  Inputs=+--
  Bus Creator : BusCreator  Inputs=2
  Demux : Demux  Outputs=2
  Gain : Gain  Gain=b
  Gain1 : Gain  Gain=d
  Rear Right Body Motion : Outport
  wires:
  Body Roll Motion/1 -> Gain1/1
  Gain1/1 -> Add/3
  Body Pitch Motion/1 -> Gain/1
  Gain/1 -> Add/2
  Body Vertical Motion/1 -> Add/1
  Demux/1 -> Bus Creator/1  "Rear Right Displacement"
  Demux/2 -> Bus Creator/2  "Rear Right Velocity"
  Add/1 -> Demux/1
  Bus Creator/1 -> Rear Right Body Motion/1  "Rear Right Body Motion"

== system All_Car_Models/Full Car Model/Full Car Model/Rear Left Wheel Suspension model/Suspension Model ==
  note: s1.s1d
  note: s2.s2d
  Wheel Motion : Inport
  Body Motion : Inport  Port=2
  " " : Sum  Inputs=+-
  " " : Sum  Inputs=+-
  Add suspention forces : Sum
  Bus Selector : BusSelector  OutputSignals=Rear Left Displacement,Rear Left Velocity
  Demux : Demux  Outputs=2
  Suspension Damping Coefficient : Lookup_n-D  NumberOfTableDimensions=1  BreakpointsForDimension1=[-10 0 10]  Table=[-10*cse 0 10*csc]  InternalRulePriority=Speed  RndMeth=Simplest  InputSameDT=on
  Suspension Spring Coefficient : Lookup_n-D  NumberOfTableDimensions=1  BreakpointsForDimension1=([0 x1 x2 2*x2])  Table=([0 ks*x1 ksstiff*(x2-x1)-(ks*x1) ksSteel*x2-(ksstiff*(x2-x1)-(ks*x1))])  InternalRulePriority=Speed  RndMeth=Simplest  InputSameDT=on
  Suspension Force : Outport
  wires:
  Bus Selector/2 -> " "/2  "<Rear Left Velocity>"
  " "/1 -> Suspension Spring Coefficient/1  "s1-s2"
  Bus Selector/1 -> " "/2  "<Rear Left Displacement>"
  Suspension Damping Coefficient/1 -> Add suspention forces/2
  Suspension Spring Coefficient/1 -> Add suspention forces/1
  Demux/1 -> " "/1  "Left Rear Wheel Displacment"
  Body Motion/1 -> Bus Selector/1
  " "/1 -> Suspension Damping Coefficient/1  "s1d-s2d"
  Wheel Motion/1 -> Demux/1
  Demux/2 -> " "/1  "Left Rear Wheel Velociy"
  Add suspention forces/1 -> Suspension Force/1

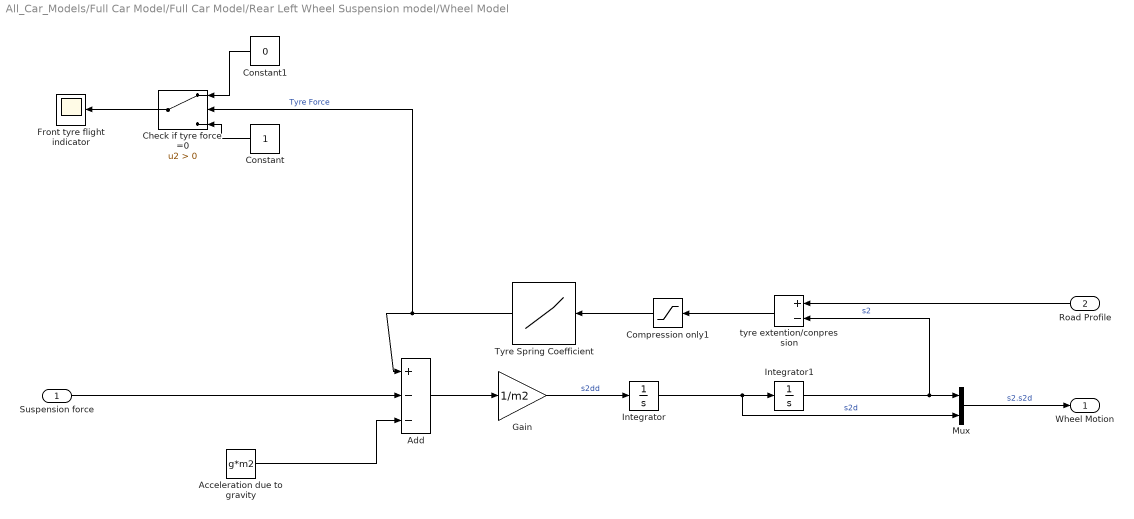
== system All_Car_Models/Full Car Model/Full Car Model/Rear Left Wheel Suspension model/Wheel Model ==
  Suspension force : Inport
  Road Profile : Inport  Port=2
  Acceleration due to gravity : Constant  Value=g*m2
  Add : Sum  Inputs=+--
  Check if tyre force =0 : Switch  Criteria=u2 > Threshold
  Compression only1 : Saturate  UpperLimit=inf  LowerLimit=0
  Constant : Constant
  Constant1 : Constant  Value=0
  Front tyre flight indicator : Scope
  Gain : Gain  Gain=1/m2
  Integrator : Integrator
  Integrator1 : Integrator  InitialCondition=-2.03e-02
  Mux : Mux  Inputs=2
  Tyre Spring Coefficient : Lookup_n-D  NumberOfTableDimensions=1  BreakpointsForDimension1=[0 xt_Lim 2*xt_Lim]  Table=[0 xt_Lim*kt ksSteel*2*xt_Lim]  InternalRulePriority=Speed  RndMeth=Simplest  InputSameDT=on
  tyre extention/conpression : Sum  Inputs=+-
  Wheel Motion : Outport
  wires:
  Integrator1/1 -> Mux/1, tyre extention/conpression/2  "s2"
  Integrator/1 -> Mux/2, Integrator1/1  "s2d"
  Add/1 -> Gain/1
  Tyre Spring Coefficient/1 -> Check if tyre force =0/2, Add/1  "Tyre Force"
  Road Profile/1 -> tyre extention/conpression/1
  Mux/1 -> Wheel Motion/1  "s2.s2d"
  Acceleration due to gravity/1 -> Add/3
  Suspension force/1 -> Add/2
  Gain/1 -> Integrator/1  "s2dd"
  tyre extention/conpression/1 -> Compression only1/1
  Compression only1/1 -> Tyre Spring Coefficient/1
  Check if tyre force =0/1 -> Front tyre flight indicator/1
  Constant1/1 -> Check if tyre force =0/1
  Constant/1 -> Check if tyre force =0/3

== system All_Car_Models/Full Car Model/Full Car Model/Rear Right Suspension model/Suspention Model ==
  note: s1.s1d
  note: s2.s2d
  Wheel Motion : Inport
  Body Motion : Inport  Port=2
  " " : Sum  Inputs=+-
  " " : Sum  Inputs=+-
  Add Suspension forces : Sum
  Bus Selector : BusSelector  OutputSignals=Rear Right Displacement,Rear Right Velocity
  Demux : Demux  Outputs=2
  Suspension Damping Coefficient : Lookup_n-D  NumberOfTableDimensions=1  BreakpointsForDimension1=[-10 0 10]  Table=[-10*cse 0 10*csc]  InternalRulePriority=Speed  RndMeth=Simplest  InputSameDT=on
  Suspension Spring Coefficient : Lookup_n-D  NumberOfTableDimensions=1  BreakpointsForDimension1=([0 x1 x2 2*x2])  Table=([0 ks*x1 ksstiff*(x2-x1)-(ks*x1) ksSteel*x2-(ksstiff*(x2-x1)-(ks*x1))])  InternalRulePriority=Speed  RndMeth=Simplest  InputSameDT=on
  Suspension Force : Outport
  wires:
  Bus Selector/2 -> " "/2  "<Rear Right Velocity>"
  " "/1 -> Suspension Spring Coefficient/1  "s1-s2"
  Bus Selector/1 -> " "/2  "<Rear Right Displacement>"
  Suspension Damping Coefficient/1 -> Add Suspension forces/2
  Suspension Spring Coefficient/1 -> Add Suspension forces/1
  Demux/1 -> " "/1  "Rear Right Wheel Displacment"
  Demux/2 -> " "/1  "Rear Right Wheel Velocity"
  Body Motion/1 -> Bus Selector/1
  " "/1 -> Suspension Damping Coefficient/1  "s1d-s2d"
  Add Suspension forces/1 -> Suspension Force/1
  Wheel Motion/1 -> Demux/1

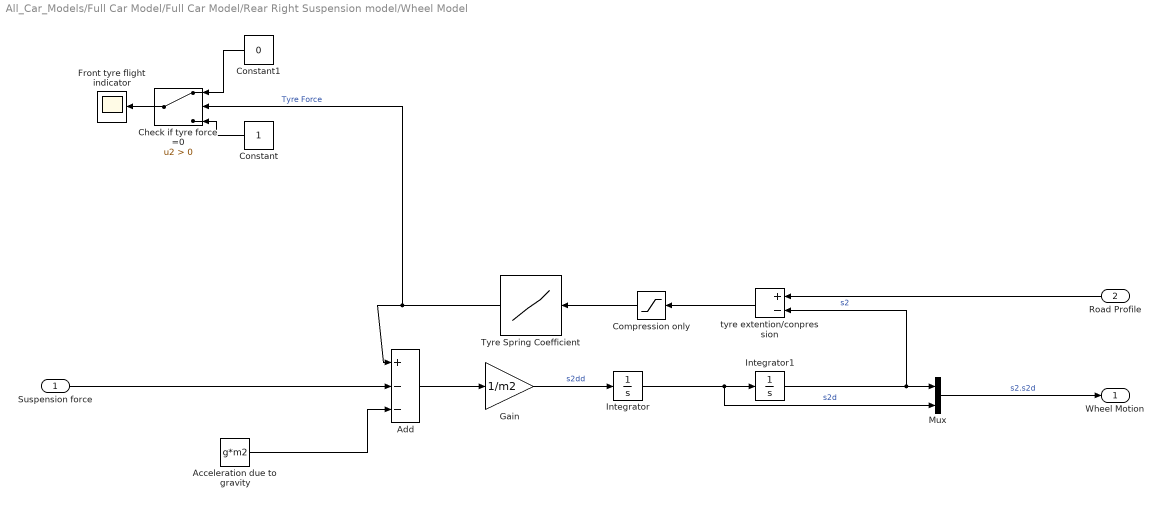
== system All_Car_Models/Full Car Model/Full Car Model/Rear Right Suspension model/Wheel Model ==
  Suspension force : Inport
  Road Profile : Inport  Port=2
  Acceleration due to gravity : Constant  Value=g*m2
  Add : Sum  Inputs=+--
  Check if tyre force =0 : Switch  Criteria=u2 > Threshold
  Compression only : Saturate  UpperLimit=inf  LowerLimit=0
  Constant : Constant
  Constant1 : Constant  Value=0
  Front tyre flight indicator : Scope
  Gain : Gain  Gain=1/m2
  Integrator : Integrator
  Integrator1 : Integrator  InitialCondition=-1.56e-02
  Mux : Mux  Inputs=2
  Tyre Spring Coefficient : Lookup_n-D  NumberOfTableDimensions=1  BreakpointsForDimension1=[0 xt_Lim 2*xt_Lim]  Table=[0 xt_Lim*kt ksSteel*2*xt_Lim]  InternalRulePriority=Speed  RndMeth=Simplest  InputSameDT=on
  tyre extention/conpression : Sum  Inputs=+-
  Wheel Motion : Outport
  wires:
  Integrator1/1 -> Mux/1, tyre extention/conpression/2  "s2"
  Integrator/1 -> Mux/2, Integrator1/1  "s2d"
  Add/1 -> Gain/1
  Tyre Spring Coefficient/1 -> Check if tyre force =0/2, Add/1  "Tyre Force"
  Road Profile/1 -> tyre extention/conpression/1
  Mux/1 -> Wheel Motion/1  "s2.s2d"
  Acceleration due to gravity/1 -> Add/3
  Suspension force/1 -> Add/2
  Gain/1 -> Integrator/1  "s2dd"
  tyre extention/conpression/1 -> Compression only/1
  Compression only/1 -> Tyre Spring Coefficient/1
  Check if tyre force =0/1 -> Front tyre flight indicator/1
  Constant1/1 -> Check if tyre force =0/1
  Constant/1 -> Check if tyre force =0/3

== system All_Car_Models/Half Car Model/1//2 Car Model/Front Wheel Suspention model/Suspention Model ==
  note: s1.s1d
  note: s2.s2d
  Wheel Motion : Inport
  Body Motion : Inport  Port=2
  " " : Sum  Inputs=+-
  " " : Sum  Inputs=+-
  Add suspention forces : Sum
  Demux : Demux  Outputs=2
  Demux1 : Demux  Outputs=2
  Suspension Stiffness : Lookup_n-D  NumberOfTableDimensions=1  BreakpointsForDimension1=[-x2*2 -x1 x1 x2*2]  Table=[-(ksstiff*(2*x2-x1)+ks*x1) -x1*ks x1*ks (ksstiff*(2*x2-x1)+ks*x1)]  InternalRulePriority=Speed  RndMeth=Simplest  InputSameDT=on
  Suspention Damping Coefficient : Lookup_n-D  NumberOfTableDimensions=1  BreakpointsForDimension1=[-10 0 10]  Table=[-10*cse 0 10*csc]  InternalRulePriority=Speed  RndMeth=Simplest  InputSameDT=on
  Suspention Force : Outport
  wires:
  Demux1/2 -> " "/2
  " "/1 -> Suspension Stiffness/1  "s1-s2"
  Demux1/1 -> " "/2
  Suspention Damping Coefficient/1 -> Add suspention forces/2
  Demux/1 -> " "/1
  Demux/2 -> " "/1
  Body Motion/1 -> Demux1/1
  " "/1 -> Suspention Damping Coefficient/1  "s1d-s2d"
  Add suspention forces/1 -> Suspention Force/1
  Wheel Motion/1 -> Demux/1
  Suspension Stiffness/1 -> Add suspention forces/1

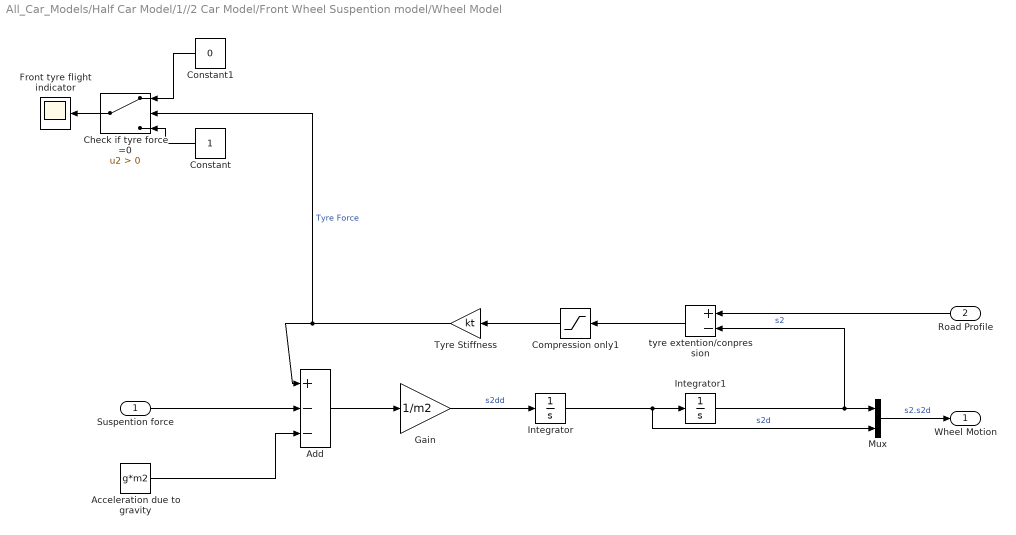
== system All_Car_Models/Half Car Model/1//2 Car Model/Front Wheel Suspention model/Wheel Model ==
  Suspention force : Inport
  Road Profile : Inport  Port=2
  Acceleration due to gravity : Constant  Value=g*m2
  Add : Sum  Inputs=+--
  Check if tyre force =0 : Switch  Criteria=u2 > Threshold
  Compression only1 : Saturate  UpperLimit=inf  LowerLimit=0
  Constant : Constant
  Constant1 : Constant  Value=0
  Front tyre flight indicator : Scope
  Gain : Gain  Gain=1/m2
  Integrator : Integrator
  Integrator1 : Integrator  InitialCondition=-0.02
  Mux : Mux  Inputs=2
  Tyre Stiffness : Gain  Gain=kt
  tyre extention/conpression : Sum  Inputs=+-
  Wheel Motion : Outport
  wires:
  Integrator1/1 -> Mux/1, tyre extention/conpression/2  "s2"
  Integrator/1 -> Mux/2, Integrator1/1  "s2d"
  Add/1 -> Gain/1
  Tyre Stiffness/1 -> Check if tyre force =0/2, Add/1  "Tyre Force"
  Road Profile/1 -> tyre extention/conpression/1
  Mux/1 -> Wheel Motion/1  "s2.s2d"
  Acceleration due to gravity/1 -> Add/3
  Suspention force/1 -> Add/2
  Gain/1 -> Integrator/1  "s2dd"
  tyre extention/conpression/1 -> Compression only1/1
  Compression only1/1 -> Tyre Stiffness/1
  Check if tyre force =0/1 -> Front tyre flight indicator/1
  Constant1/1 -> Check if tyre force =0/1
  Constant/1 -> Check if tyre force =0/3

== system All_Car_Models/Half Car Model/1//2 Car Model/Rear Wheel Suspention model/Suspention Model ==
  note: s1.s1d
  note: s2.s2d
  Wheel Motion : Inport
  Body Motion : Inport  Port=2
  " " : Sum  Inputs=+-
  " " : Sum  Inputs=+-
  Add suspention forces : Sum
  Demux : Demux  Outputs=2
  Demux1 : Demux  Outputs=2
  Suspension Stiffness : Lookup_n-D  NumberOfTableDimensions=1  BreakpointsForDimension1=[-x2*2 -x1 x1 x2*2]  Table=[-(ksstiff*(2*x2-x1)+ks*x1) -x1*ks x1*ks (ksstiff*(2*x2-x1)+ks*x1)]  InternalRulePriority=Speed  RndMeth=Simplest  InputSameDT=on
  Suspention Damping Coefficient : Lookup_n-D  NumberOfTableDimensions=1  BreakpointsForDimension1=[-10 0 10]  Table=[-10*cse 0 10*csc]  InternalRulePriority=Speed  RndMeth=Simplest  InputSameDT=on
  Suspention Force : Outport
  wires:
  Demux1/2 -> " "/2  "s1d"
  " "/1 -> Suspension Stiffness/1  "s1-s2"
  Demux1/1 -> " "/2  "s1"
  Suspention Damping Coefficient/1 -> Add suspention forces/2
  Suspension Stiffness/1 -> Add suspention forces/1
  Demux/1 -> " "/1  "s2"
  Demux/2 -> " "/1  "s2d"
  Body Motion/1 -> Demux1/1
  " "/1 -> Suspention Damping Coefficient/1  "s1d-s2d"
  Add suspention forces/1 -> Suspention Force/1
  Wheel Motion/1 -> Demux/1

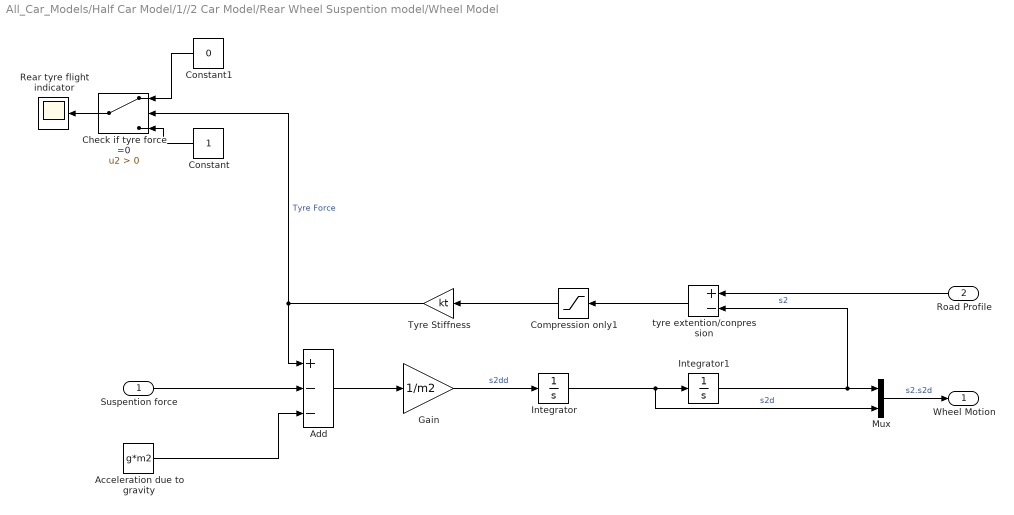
== system All_Car_Models/Half Car Model/1//2 Car Model/Rear Wheel Suspention model/Wheel Model ==
  Suspention force : Inport
  Road Profile : Inport  Port=2
  Acceleration due to gravity : Constant  Value=g*m2
  Add : Sum  Inputs=+--
  Check if tyre force =0 : Switch  Criteria=u2 > Threshold
  Compression only1 : Saturate  UpperLimit=inf  LowerLimit=0
  Constant : Constant
  Constant1 : Constant  Value=0
  Gain : Gain  Gain=1/m2
  Integrator : Integrator
  Integrator1 : Integrator  InitialCondition=-0.018
  Mux : Mux  Inputs=2
  Rear tyre flight indicator : Scope
  Tyre Stiffness : Gain  Gain=kt
  tyre extention/conpression : Sum  Inputs=+-
  Wheel Motion : Outport
  wires:
  Integrator1/1 -> tyre extention/conpression/2, Mux/1  "s2"
  Integrator/1 -> Mux/2, Integrator1/1  "s2d"
  Add/1 -> Gain/1
  Road Profile/1 -> tyre extention/conpression/1
  Mux/1 -> Wheel Motion/1  "s2.s2d"
  Acceleration due to gravity/1 -> Add/3
  Suspention force/1 -> Add/2
  Gain/1 -> Integrator/1  "s2dd"
  tyre extention/conpression/1 -> Compression only1/1
  Constant/1 -> Check if tyre force =0/3
  Check if tyre force =0/1 -> Rear tyre flight indicator/1
  Constant1/1 -> Check if tyre force =0/1
  Compression only1/1 -> Tyre Stiffness/1
  Tyre Stiffness/1 -> Add/1, Check if tyre force =0/2  "Tyre Force"

== system All_Car_Models/Half Car Model/1//2 Car Model Improved/Front Wheel Suspension model/Suspension Model ==
  note: s1.s1d
  note: s2.s2d
  Wheel Motion : Inport
  Body Motion : Inport  Port=2
  " " : Sum  Inputs=+-
  " " : Sum  Inputs=+-
  Add Suspension forces : Sum
  Demux : Demux  Outputs=2
  Demux1 : Demux  Outputs=2
  Suspension Damping Coefficient : Lookup_n-D  NumberOfTableDimensions=1  BreakpointsForDimension1=[-10 0 10]  Table=[-10*cse 0 10*csc]  InternalRulePriority=Speed  RndMeth=Simplest  InputSameDT=on
  Suspension Spring Coefficient : Lookup_n-D  NumberOfTableDimensions=1  BreakpointsForDimension1=([0 x1 x2 2*x2])  Table=([0 ks*x1 ksstiff*(x2-x1)-(ks*x1) ksSteel*x2-(ksstiff*(x2-x1)-(ks*x1))])  InternalRulePriority=Speed  RndMeth=Simplest  InputSameDT=on
  Suspension Force : Outport
  wires:
  Demux1/2 -> " "/2
  " "/1 -> Suspension Spring Coefficient/1  "s1-s2"
  Demux1/1 -> " "/2
  Suspension Damping Coefficient/1 -> Add Suspension forces/2
  Demux/1 -> " "/1
  Demux/2 -> " "/1
  Body Motion/1 -> Demux1/1
  " "/1 -> Suspension Damping Coefficient/1  "s1d-s2d"
  Add Suspension forces/1 -> Suspension Force/1
  Wheel Motion/1 -> Demux/1
  Suspension Spring Coefficient/1 -> Add Suspension forces/1
